simulink model "Hohmann"  (R2024b)
settings: Solver=ode4  StartTime=0.0  StopTime=T_end_Hohmann  FixedStep=0.01  RelTol=1e-3
values from neighbouring files (symbols this model uses):
  A = ly*lz    (= 0.25)    [Main.m]
  CD = 2.2    [Main.m]
  deltat_onOP = m_c0*deltaVx/Total_max_thrust    [Main.m]
  deltaVx = omega_chaser/4*Pos0(3)    [Main.m]
  deltax = 3*pi/omega_chaser*deltaVx    [Main.m]
  deltax_FD = 0    [Main.m]
  KF = (Uon-Uoff)/(1-exp(-deltat_on/tau))    [Main.m]
  lambda = 0.5    [Main.m]
  m_c0 = 50    [Main.m]
  omega_target = (mu/r_target^3)^0.5    (= 0.00113136572666)    [Main.m]
  Pos0 = [x0 y0 z0]'    [Main.m]
  rho = 1*10^(-12)    (= 1e-12)    [Main.m]
  S = 0.9    [Main.m]
  T_1fire = abs(deltax_FD)/x0_dot    [Main.m]
  T_2fire = T_1fire+ T_Hohmann/2    [Main.m]
  tau = -ton/(log(1-(Uon-Uoff)/(Tmax*kf)))    [Main.m]
  Tmax = 1    [Main.m]
  Uoff = 0.7    [Main.m]
  Uon = 1    [Main.m]
  Vel0 = [x0_dot y0_dot z0_dot]'    [Main.m]
  Vx = omega_target*r_target    (= 7668.56094333)    [Main.m]
  x0 = -10*10^3    (= -10000)    [Main.m]
settings Model: Creator=aless  LastModifiedBy=aless

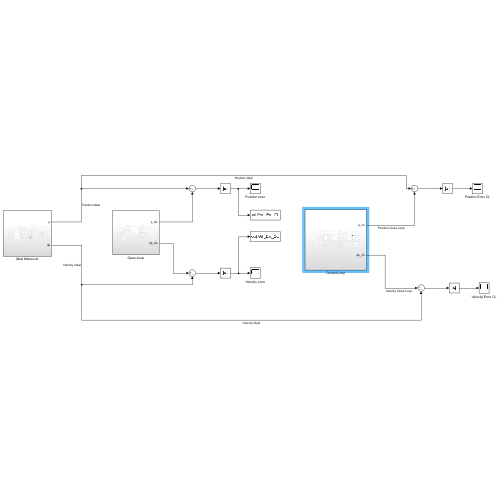
[thumbnail: Simulink's stored preview of the top-level diagram]
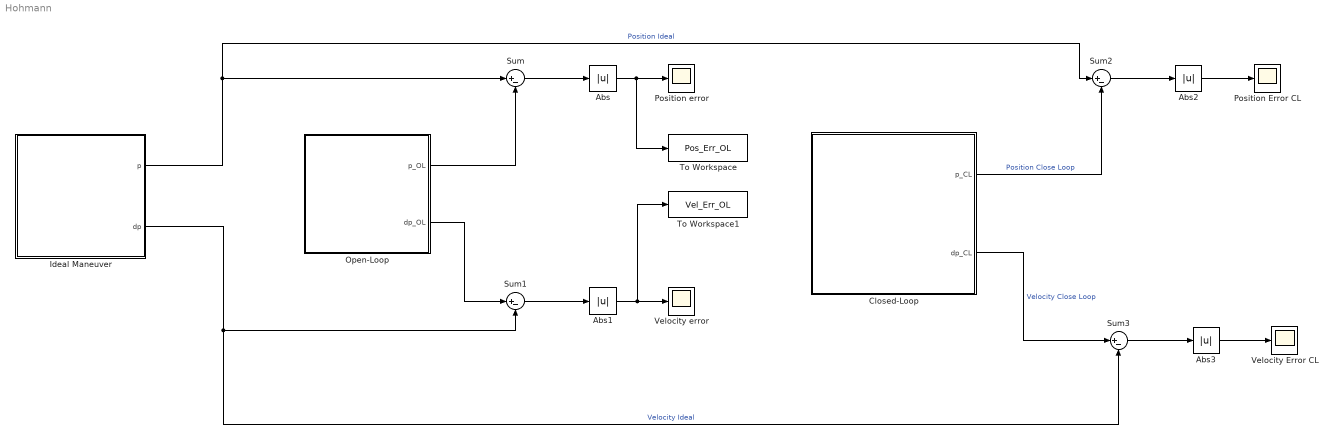
== system Hohmann ==
  Abs{,1..3} (4 alike) : Abs  SaturateOnIntegerOverflow=off
  Closed-Loop : Subsystem
  Ideal Maneuver : Subsystem
  Open-Loop : Subsystem
  Position Error CL : Scope
  Position error : Scope
  Sum{,1..3} (4 alike) : Sum  Inputs=|+-
  To Workspace : ToWorkspace  VariableName=Pos_Err_OL  SaveFormat=Timeseries  SampleTime=-1
  To Workspace1 : ToWorkspace  VariableName=Vel_Err_OL  SaveFormat=Timeseries  SampleTime=-1
  Velocity Error CL : Scope
  Velocity error : Scope
  wires:
  Sum/1 -> Abs/1
  Ideal Maneuver/2(dp) -> Sum3/2, Sum1/2  "Velocity Ideal"
  Sum2/1 -> Abs2/1
  Closed-Loop/1(p_CL) -> Sum2/2  "Position Close Loop"
  Open-Loop/2(dp_OL) -> Sum1/1
  Open-Loop/1(p_OL) -> Sum/2
  Abs2/1 -> Position Error CL/1
  Sum1/1 -> Abs1/1
  Abs3/1 -> Velocity Error CL/1
  Sum3/1 -> Abs3/1
  Abs1/1 -> To Workspace1/1, Velocity error/1
  Closed-Loop/2(dp_CL) -> Sum3/1  "Velocity Close Loop"
  Abs/1 -> To Workspace/1, Position error/1
  Ideal Maneuver/1(p) -> Sum2/1, Sum/1  "Position Ideal"

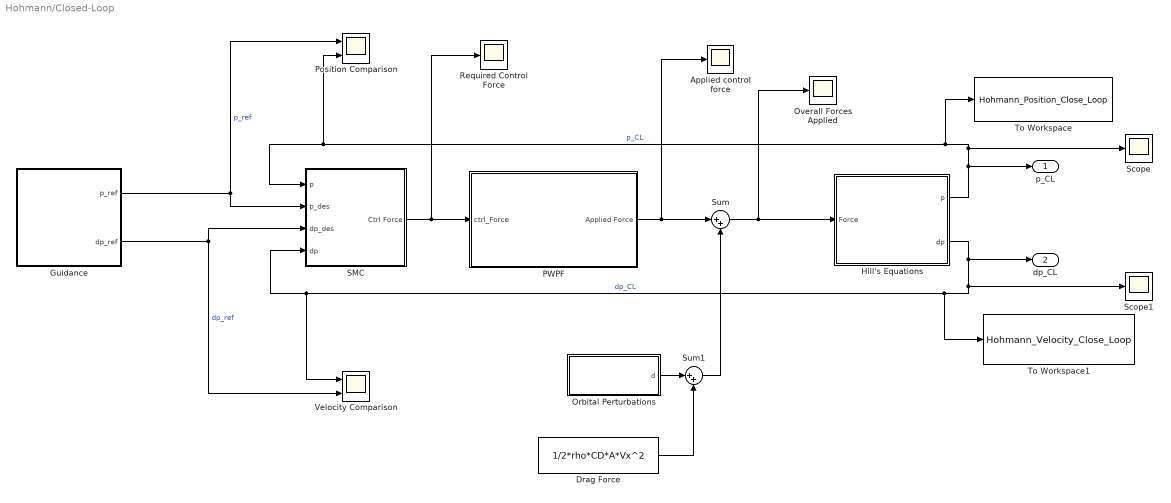
== system Hohmann/Closed-Loop ==
  Applied control force : Scope
  Drag Force : Constant  Value=1/2*rho*CD*A*Vx^2
  Guidance : Subsystem
  Hill's Equations : Subsystem
  Orbital Perturbations : Subsystem
  Overall Forces Applied : Scope
  PWPF : Subsystem
  Position Comparison : Scope  NumInputPorts=2
  Required Control Force : Scope
  SMC : Subsystem
  Scope : Scope
  Scope1 : Scope
  Sum : Sum  Inputs=|++
  Sum1 : Sum  Inputs=|++
  To Workspace : ToWorkspace  VariableName=Hohmann_Position_Close_Loop  SaveFormat=Timeseries  SampleTime=-1
  To Workspace1 : ToWorkspace  VariableName=Hohmann_Velocity_Close_Loop  SaveFormat=Timeseries  SampleTime=-1
  Velocity Comparison : Scope  NumInputPorts=2
  p_CL : Outport
  dp_CL : Outport  Port=2
  wires:
  Guidance/2(dp_ref) -> Velocity Comparison/2, SMC/3(dp_des)  "dp_ref"
  Hill's Equations/2(dp) -> To Workspace1/1, Velocity Comparison/1, SMC/4(dp), Scope1/1, dp_CL/1  "dp_CL"
  Guidance/1(p_ref) -> SMC/2(p_des), Position Comparison/1  "p_ref"
  Hill's Equations/1(p) -> p_CL/1, To Workspace/1, Position Comparison/2, SMC/1(p), Scope/1  "p_CL"
  SMC/1(Ctrl Force) -> PWPF/1(ctrl_Force), Required Control Force/1
  PWPF/1(Applied Force) -> Applied control force/1, Sum/1
  Sum/1 -> Overall Forces Applied/1, Hill's Equations/1(Force)
  Orbital Perturbations/1(d) -> Sum1/1
  Drag Force/1 -> Sum1/2
  Sum1/1 -> Sum/2

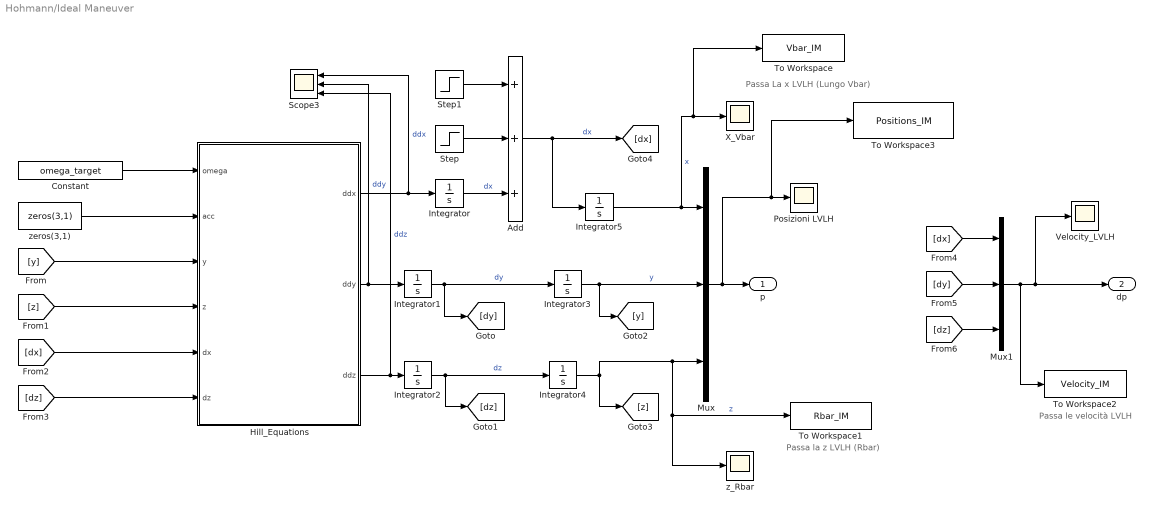
== system Hohmann/Ideal Maneuver ==
  note: Passa La x LVLH (Lungo Vbar)
  note: Passa le velocità LVLH
  note: Passa la z LVLH (Rbar)
  Add : Sum  Inputs=+++
  Constant : Constant  Value=omega_target
  Hill_Equations : MATLAB Function  TreatAsAtomicUnit=on
  Integrator : Integrator  InitialCondition=Vel0(1)
  Integrator1 : Integrator  InitialCondition=Vel0(2)
  Integrator2 : Integrator  InitialCondition=Vel0(3)
  Integrator3 : Integrator  InitialCondition=Pos0(2)
  Integrator4 : Integrator  InitialCondition=Pos0(3)
  Integrator5 : Integrator  InitialCondition=-(deltax+3000)
  Mux : Mux  Inputs=3
  Mux1 : Mux  Inputs=3
  Posizioni LVLH : Scope
  Scope3 : Scope  NumInputPorts=3
  Step : Step  Time=T_1fire  After=deltaVx  SampleTime=0
  Step1 : Step  Time=T_2fire  After=deltaVx  SampleTime=0
  To Workspace : ToWorkspace  VariableName=Vbar_IM  SaveFormat=Timeseries  SampleTime=-1
  To Workspace1 : ToWorkspace  VariableName=Rbar_IM  SaveFormat=Timeseries  SampleTime=-1
  To Workspace2 : ToWorkspace  VariableName=Velocity_IM  SaveFormat=Timeseries  SampleTime=-1
  To Workspace3 : ToWorkspace  VariableName=Positions_IM  SaveFormat=Timeseries  SampleTime=-1
  Velocity_LVLH : Scope
  X_Vbar : Scope
  z_Rbar : Scope
  zeros(3,1) : Constant  Value=zeros(3,1)
  p : Outport
  dp : Outport  Port=2
  wires:
  Add/1 -> Integrator5/1, [dx]  "dx"
  Integrator5/1 -> To Workspace/1, X_Vbar/1, Mux/1  "x"
  Integrator/1 -> Add/3  "dx"
  Integrator2/1 -> [dz], Integrator4/1  "dz"
  Integrator1/1 -> [dy], Integrator3/1  "dy"
  Hill_Equations/2(ddy) -> Scope3/2, Integrator1/1  "ddy"
  Mux/1 -> To Workspace3/1, Posizioni LVLH/1, p/1
  Constant/1 -> Hill_Equations/1(omega)
  [dz] -> Hill_Equations/6(dz)
  [y] -> Hill_Equations/3(y)
  zeros(3,1)/1 -> Hill_Equations/2(acc)
  [z] -> Hill_Equations/4(z)
  [dx] -> Hill_Equations/5(dx)
  Integrator4/1 -> To Workspace1/1, z_Rbar/1, Mux/3, [z]  "z"
  Integrator3/1 -> [y], Mux/2  "y"
  Hill_Equations/3(ddz) -> Scope3/3, Integrator2/1  "ddz"
  Hill_Equations/1(ddx) -> Scope3/1, Integrator/1  "ddx"
  [dx] -> Mux1/1
  [dy] -> Mux1/2
  [dz] -> Mux1/3
  Mux1/1 -> To Workspace2/1, Velocity_LVLH/1, dp/1
  Step/1 -> Add/2
  Step1/1 -> Add/1

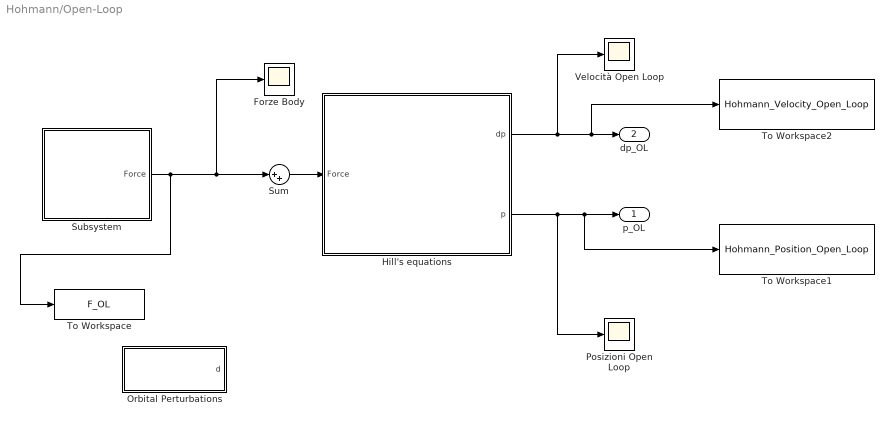
== system Hohmann/Open-Loop ==
  Forze Body : Scope
  Hill's equations : Subsystem
  Orbital Perturbations : Subsystem
  Posizioni Open Loop : Scope
  Subsystem : Subsystem
  Sum : Sum  Inputs=|++
  To Workspace : ToWorkspace  VariableName=F_OL  SaveFormat=Timeseries  SampleTime=-1
  To Workspace1 : ToWorkspace  VariableName=Hohmann_Position_Open_Loop  SaveFormat=Timeseries  SampleTime=-1
  To Workspace2 : ToWorkspace  VariableName=Hohmann_Velocity_Open_Loop  SaveFormat=Timeseries  SampleTime=-1
  Velocità Open Loop : Scope
  p_OL : Outport
  dp_OL : Outport  Port=2
  wires:
  Hill's equations/2(p) -> To Workspace1/1, p_OL/1, Posizioni Open Loop/1
  Hill's equations/1(dp) -> dp_OL/1, To Workspace2/1, Velocità Open Loop/1
  Subsystem/1(Force) -> To Workspace/1, Sum/1, Forze Body/1
  Sum/1 -> Hill's equations/1(Force)

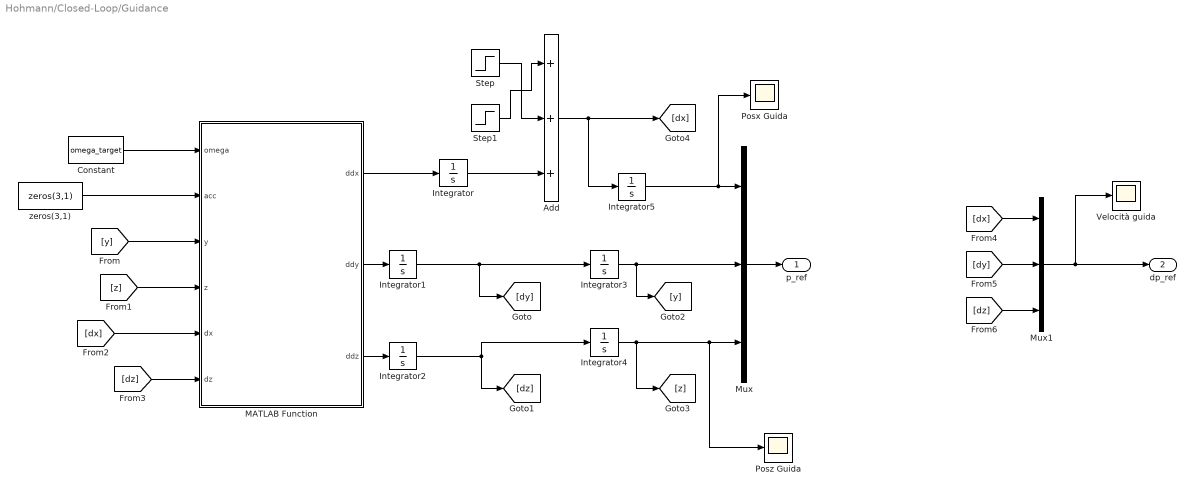
== system Hohmann/Closed-Loop/Guidance ==
  Add : Sum  Inputs=+++
  Constant : Constant  Value=omega_target
  Integrator : Integrator  InitialCondition=Vel0(1)
  Integrator1 : Integrator  InitialCondition=Vel0(2)
  Integrator2 : Integrator  InitialCondition=Vel0(3)
  Integrator3 : Integrator  InitialCondition=Pos0(2)
  Integrator4 : Integrator  InitialCondition=Pos0(3)
  Integrator5 : Integrator  InitialCondition=Pos0(1)+deltax_FD
  MATLAB Function : MATLAB Function  TreatAsAtomicUnit=on
  Mux : Mux  Inputs=3
  Mux1 : Mux  Inputs=3
  Posx Guida : Scope
  Posz Guida : Scope
  Step : Step  Time=T_1fire  After=deltaVx  SampleTime=0
  Step1 : Step  Time=T_2fire  After=deltaVx  SampleTime=0
  Velocità guida : Scope
  zeros(3,1) : Constant  Value=zeros(3,1)
  p_ref : Outport
  dp_ref : Outport  Port=2
  wires:
  Mux1/1 -> Velocità guida/1, dp_ref/1
  Mux/1 -> p_ref/1
  MATLAB Function/3(ddz) -> Integrator2/1
  Integrator/1 -> Add/3
  [y] -> MATLAB Function/3(y)
  Constant/1 -> MATLAB Function/1(omega)
  MATLAB Function/1(ddx) -> Integrator/1
  [dx] -> Mux1/1
  [z] -> MATLAB Function/4(z)
  Integrator3/1 -> [y], Mux/2
  zeros(3,1)/1 -> MATLAB Function/2(acc)
  Add/1 -> Integrator5/1, [dx]
  [dz] -> Mux1/3
  [dx] -> MATLAB Function/5(dx)
  [dz] -> MATLAB Function/6(dz)
  Integrator4/1 -> [z], Posz Guida/1, Mux/3
  Step/1 -> Add/2
  Step1/1 -> Add/1
  Integrator5/1 -> Posx Guida/1, Mux/1
  Integrator1/1 -> [dy], Integrator3/1
  Integrator2/1 -> [dz], Integrator4/1
  MATLAB Function/2(ddy) -> Integrator1/1
  [dy] -> Mux1/2

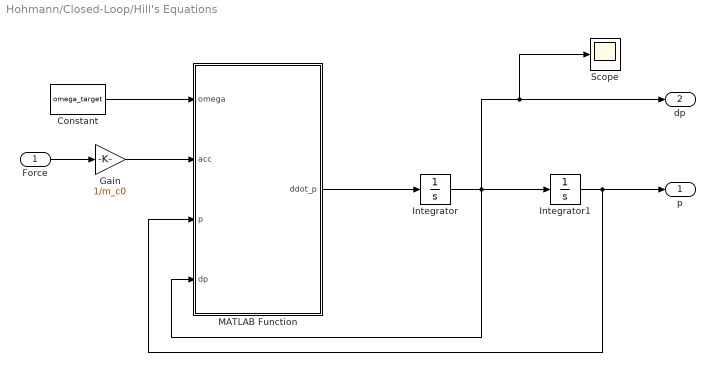
== system Hohmann/Closed-Loop/Hill's Equations ==
  Force : Inport
  Constant : Constant  Value=omega_target
  Gain : Gain  Gain=1/m_c0
  Integrator : Integrator  InitialCondition=Vel0'
  Integrator1 : Integrator  InitialCondition=x0
  MATLAB Function : MATLAB Function  TreatAsAtomicUnit=on
  Scope : Scope
  p : Outport
  dp : Outport  Port=2
  wires:
  Gain/1 -> MATLAB Function/2(acc)
  Force/1 -> Gain/1
  Integrator1/1 -> p/1, MATLAB Function/3(p)
  MATLAB Function/1(ddot_p) -> Integrator/1
  Integrator/1 -> dp/1, Scope/1, MATLAB Function/4(dp), Integrator1/1
  Constant/1 -> MATLAB Function/1(omega)

== system Hohmann/Closed-Loop/Orbital Perturbations ==
  Add : Sum
  Constant : Constant  Value=[0.01 0.01 0.01]
  Mux : Mux  Inputs=3
  Random Number : RandomNumber  Variance=(0.00001)^2  Seed=1  SampleTime=1
  Random Number1 : RandomNumber  Variance=(0.00001)^2  Seed=765  SampleTime=1
  Random Number2 : RandomNumber  Variance=(0.00001)^2  Seed=6  SampleTime=1
  d : Outport
  wires:
  Add/1 -> d/1
  Constant/1 -> Add/1
  Mux/1 -> Add/2
  Random Number2/1 -> Mux/3
  Random Number1/1 -> Mux/2
  Random Number/1 -> Mux/1

== system Hohmann/Closed-Loop/PWPF ==
  ctrl_Force : Inport
  Demux : Demux  Outputs=3
  Mux : Mux  Inputs=3
  Subsystem : Subsystem
  Subsystem1 : Subsystem
  Subsystem2 : Subsystem
  Applied Force : Outport
  wires:
  ctrl_Force/1 -> Demux/1
  Demux/1 -> Subsystem/1(Ctrl_Force_x)
  Demux/2 -> Subsystem1/1(Ctrl_Force_y)
  Demux/3 -> Subsystem2/1(Ctrl_Force_z)
  Subsystem/1(Applied_Force_x) -> Mux/1
  Mux/1 -> Applied Force/1
  Subsystem1/1(Applied_Force_y) -> Mux/2
  Subsystem2/1(Applied_Force_z) -> Mux/3

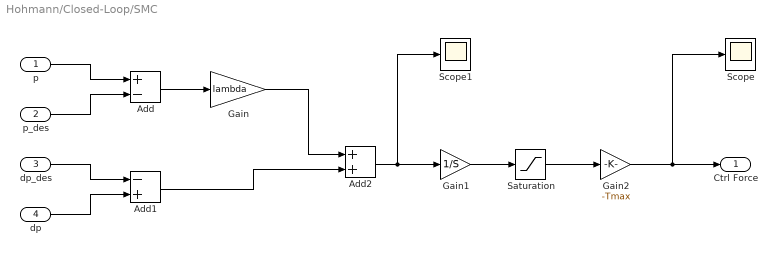
== system Hohmann/Closed-Loop/SMC ==
  p : Inport
  p_des : Inport  Port=2
  dp_des : Inport  Port=3
  dp : Inport  Port=4
  Add : Sum  Inputs=+-
  Add1 : Sum  Inputs=-+
  Add2 : Sum
  Gain : Gain  Gain=lambda
  Gain1 : Gain  Gain=1/S
  Gain2 : Gain  Gain=-Tmax
  Saturation : Saturate  UpperLimit=1  LowerLimit=-1
  Scope : Scope
  Scope1 : Scope
  Ctrl Force : Outport
  wires:
  p_des/1 -> Add/2
  p/1 -> Add/1
  dp_des/1 -> Add1/1
  dp/1 -> Add1/2
  Add/1 -> Gain/1
  Gain/1 -> Add2/1
  Add1/1 -> Add2/2
  Add2/1 -> Scope1/1, Gain1/1
  Gain1/1 -> Saturation/1
  Saturation/1 -> Gain2/1
  Gain2/1 -> Scope/1, Ctrl Force/1

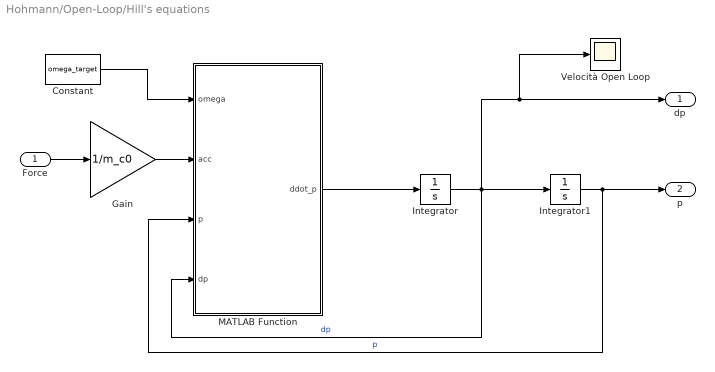
== system Hohmann/Open-Loop/Hill's equations ==
  Force : Inport
  Constant : Constant  Value=omega_target
  Gain : Gain  Gain=1/m_c0
  Integrator : Integrator  InitialCondition=Vel0'
  Integrator1 : Integrator  InitialCondition=Pos0'
  MATLAB Function : MATLAB Function  TreatAsAtomicUnit=on
  Velocità Open Loop : Scope
  dp : Outport
  p : Outport  Port=2
  wires:
  Force/1 -> Gain/1
  Gain/1 -> MATLAB Function/2(acc)
  Constant/1 -> MATLAB Function/1(omega)
  MATLAB Function/1(ddot_p) -> Integrator/1
  Integrator/1 -> Velocità Open Loop/1, dp/1, MATLAB Function/4(dp), Integrator1/1  "dp"
  Integrator1/1 -> p/1, MATLAB Function/3(p)  "p"

== system Hohmann/Open-Loop/Orbital Perturbations ==
  Add : Sum
  Constant : Constant  Value=[1e-5 0 0]
  Mux : Mux  Inputs=3
  Random Number : RandomNumber  Variance=(1e-8)^2  Seed=1  SampleTime=0.1
  Random Number1 : RandomNumber  Variance=(1e-8)^2  Seed=765  SampleTime=0.1
  Random Number2 : RandomNumber  Variance=(1e-8)^2  Seed=6  SampleTime=0.1
  d : Outport
  wires:
  Add/1 -> d/1
  Constant/1 -> Add/1
  Mux/1 -> Add/2
  Random Number2/1 -> Mux/3
  Random Number1/1 -> Mux/2
  Random Number/1 -> Mux/1

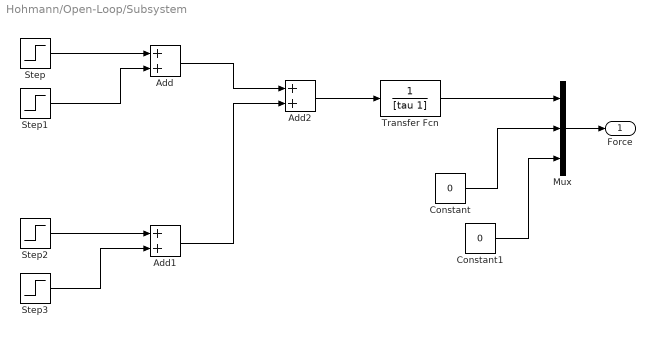
== system Hohmann/Open-Loop/Subsystem ==
  Add : Sum
  Add1 : Sum
  Add2 : Sum
  Constant : Constant  Value=0
  Constant1 : Constant  Value=0
  Mux : Mux  Inputs=3
  Step : Step  Time=T_1fire-deltat_onOP/2  After=Tmax  SampleTime=0
  Step1 : Step  Time=T_1fire+deltat_onOP/2  After=-Tmax  SampleTime=0
  Step2 : Step  Time=T_2fire-deltat_onOP/2  After=Tmax  SampleTime=0
  Step3 : Step  Time=T_2fire+deltat_onOP/2  After=-Tmax  SampleTime=0
  Transfer Fcn : TransferFcn  Denominator=[tau 1]
  Force : Outport
  wires:
  Step/1 -> Add/1
  Step1/1 -> Add/2
  Step2/1 -> Add1/1
  Step3/1 -> Add1/2
  Add/1 -> Add2/1
  Add1/1 -> Add2/2
  Add2/1 -> Transfer Fcn/1
  Transfer Fcn/1 -> Mux/1
  Mux/1 -> Force/1
  Constant1/1 -> Mux/3
  Constant/1 -> Mux/2

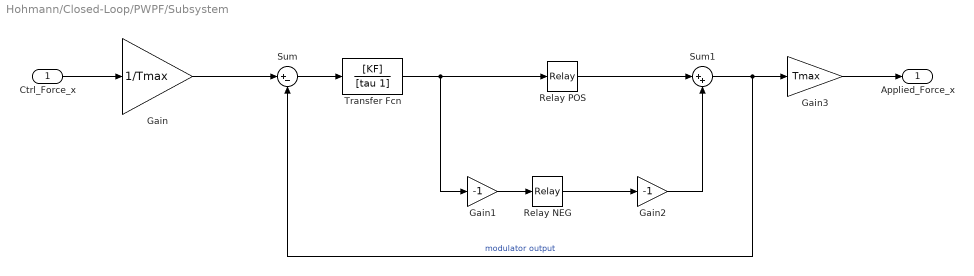
== system Hohmann/Closed-Loop/PWPF/Subsystem ==
  Ctrl_Force_x : Inport
  Gain : Gain  Gain=1/Tmax
  Gain1 : Gain  Gain=-1
  Gain2 : Gain  Gain=-1
  Gain3 : Gain  Gain=Tmax
  Relay NEG : Relay  OnSwitchValue=Uon  OffSwitchValue=Uoff
  Relay POS : Relay  OnSwitchValue=Uon  OffSwitchValue=Uoff
  Sum : Sum  Inputs=|+-
  Sum1 : Sum  Inputs=|++
  Transfer Fcn : TransferFcn  Numerator=[KF]  Denominator=[tau 1]
  Applied_Force_x : Outport
  wires:
  Transfer Fcn/1 -> Relay POS/1, Gain1/1
  Gain2/1 -> Sum1/2
  Gain1/1 -> Relay NEG/1
  Sum/1 -> Transfer Fcn/1
  Sum1/1 -> Sum/2, Gain3/1  "modulator output"
  Gain/1 -> Sum/1
  Relay POS/1 -> Sum1/1
  Relay NEG/1 -> Gain2/1
  Ctrl_Force_x/1 -> Gain/1
  Gain3/1 -> Applied_Force_x/1

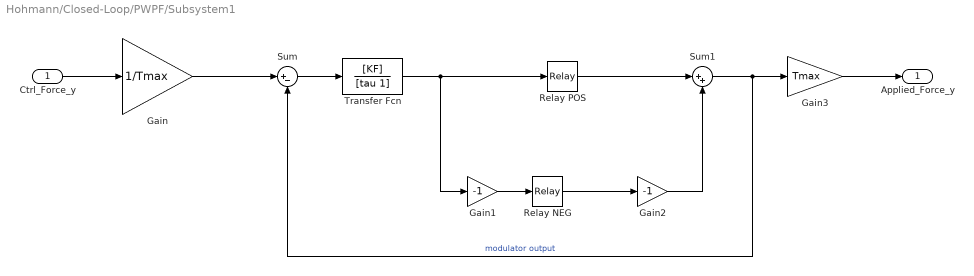
== system Hohmann/Closed-Loop/PWPF/Subsystem1 ==
  Ctrl_Force_y : Inport
  Gain : Gain  Gain=1/Tmax
  Gain1 : Gain  Gain=-1
  Gain2 : Gain  Gain=-1
  Gain3 : Gain  Gain=Tmax
  Relay NEG : Relay  OnSwitchValue=Uon  OffSwitchValue=Uoff
  Relay POS : Relay  OnSwitchValue=Uon  OffSwitchValue=Uoff
  Sum : Sum  Inputs=|+-
  Sum1 : Sum  Inputs=|++
  Transfer Fcn : TransferFcn  Numerator=[KF]  Denominator=[tau 1]
  Applied_Force_y : Outport
  wires:
  Transfer Fcn/1 -> Relay POS/1, Gain1/1
  Gain2/1 -> Sum1/2
  Gain1/1 -> Relay NEG/1
  Sum/1 -> Transfer Fcn/1
  Sum1/1 -> Sum/2, Gain3/1  "modulator output"
  Gain/1 -> Sum/1
  Relay POS/1 -> Sum1/1
  Relay NEG/1 -> Gain2/1
  Ctrl_Force_y/1 -> Gain/1
  Gain3/1 -> Applied_Force_y/1

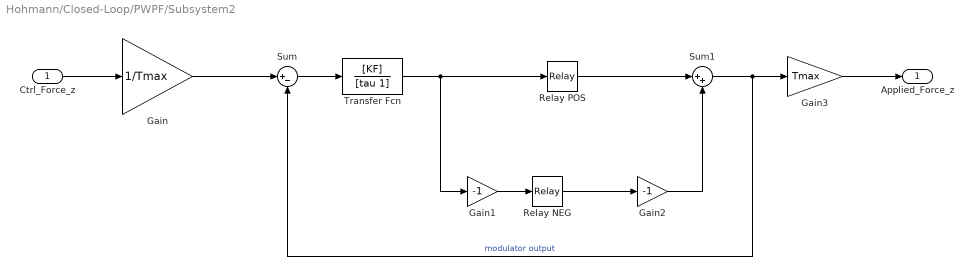
== system Hohmann/Closed-Loop/PWPF/Subsystem2 ==
  Ctrl_Force_z : Inport
  Gain : Gain  Gain=1/Tmax
  Gain1 : Gain  Gain=-1
  Gain2 : Gain  Gain=-1
  Gain3 : Gain  Gain=Tmax
  Relay NEG : Relay  OnSwitchValue=Uon  OffSwitchValue=Uoff
  Relay POS : Relay  OnSwitchValue=Uon  OffSwitchValue=Uoff
  Sum : Sum  Inputs=|+-
  Sum1 : Sum  Inputs=|++
  Transfer Fcn : TransferFcn  Numerator=[KF]  Denominator=[tau 1]
  Applied_Force_z : Outport
  wires:
  Transfer Fcn/1 -> Relay POS/1, Gain1/1
  Gain2/1 -> Sum1/2
  Gain1/1 -> Relay NEG/1
  Sum/1 -> Transfer Fcn/1
  Sum1/1 -> Sum/2, Gain3/1  "modulator output"
  Gain/1 -> Sum/1
  Relay POS/1 -> Sum1/1
  Relay NEG/1 -> Gain2/1
  Ctrl_Force_z/1 -> Gain/1
  Gain3/1 -> Applied_Force_z/1

== matlab function Hohmann/Open-Loop/Hill's equations/MATLAB Function ==
  data: omega input; ddot_p output; acc input; p input; dp input
function ddot_p = fcn(omega, acc, p, dp)

ddot_p=zeros(1,3);
x=p(1);
y=p(2);
z=p(3);
dx=dp(1);
dy=dp(2);
dz=dp(3);
ddot_p(1)=acc(1) + 2*omega*dz;
ddot_p(2)=acc(2) - omega^2*y;
ddot_p(3)=acc(3) - 2*omega*dx + 3*omega^2*z;

== matlab function Hohmann/Ideal Maneuver/Hill_Equations ==
  data: omega input; ddx output; acc input; y input; z input; dx input; dz input; ddy output; ddz output
function [ddx, ddy, ddz] = Hill_Equations(omega, acc, y, z, dx, dz)

ddx(1)=acc(1);
ddy(1)=acc(2);
ddz(1)=acc(3);

ddx = 2*omega*dz;
ddy = -omega^2*y;
ddz = 3*omega^2*z -2*omega*dx;

== matlab function Hohmann/Closed-Loop/Guidance/MATLAB Function ==
  data: omega input; ddx output; acc input; y input; z input; dx input; dz input; ddy output; ddz output
function [ddx, ddy, ddz] = fcn(omega, acc, y, z, dx, dz)

ddx(1)=acc(1);
ddy(1)=acc(2);
ddz(1)=acc(3);

ddx = 2*omega*dz;
ddy = -omega^2*y;
ddz = 3*omega^2*z -2*omega*dx;

== matlab function Hohmann/Closed-Loop/Hill's Equations/MATLAB Function ==
  data: omega input; ddot_p output; acc input; p input; dp input
function ddot_p = fcn(omega, acc, p, dp)

ddot_p=zeros(1,3);
x=p(1);
y=p(2);
z=p(3);
dx=dp(1);
dy=dp(2);
dz=dp(3);
ddot_p(1)=acc(1) + 2*omega*dz;
ddot_p(2)=acc(2) - omega^2*y;
ddot_p(3)=acc(3) - 2*omega*dx + 3*omega^2*z;
